simulink model "momentTest_th"  (R2018b)
settings: Solver=ode3  StartTime=0.0  StopTime=sim_time  FixedStep=.001  RelTol=1e-3
values from neighbouring files (symbols this model uses):
  accMag = tetherTen/mass    (= 25.8815917179)    [momentTest_ts.m]
  initPos = [path_init(1);path_init(2);path_init(3);]    [momentTest_ts.m]
  initVelTan = velMag*[cosd(initVelAng);sind(initVelAng);0]    [momentTest_ts.m]
  MOI_X = 1e5    (= 100000)    [momentTest_ts.m]
libraries: schmehlTangentRotation_ul x1, vectorNormalizer_ul x1, pathFollowingController_cl x1
settings Model: Creator=jldanie5  LastModifiedBy=jldanie5
settings DebuggingCC: BusObjectLabelMismatch=none  UnderSpecifiedDimensionMsg=warning

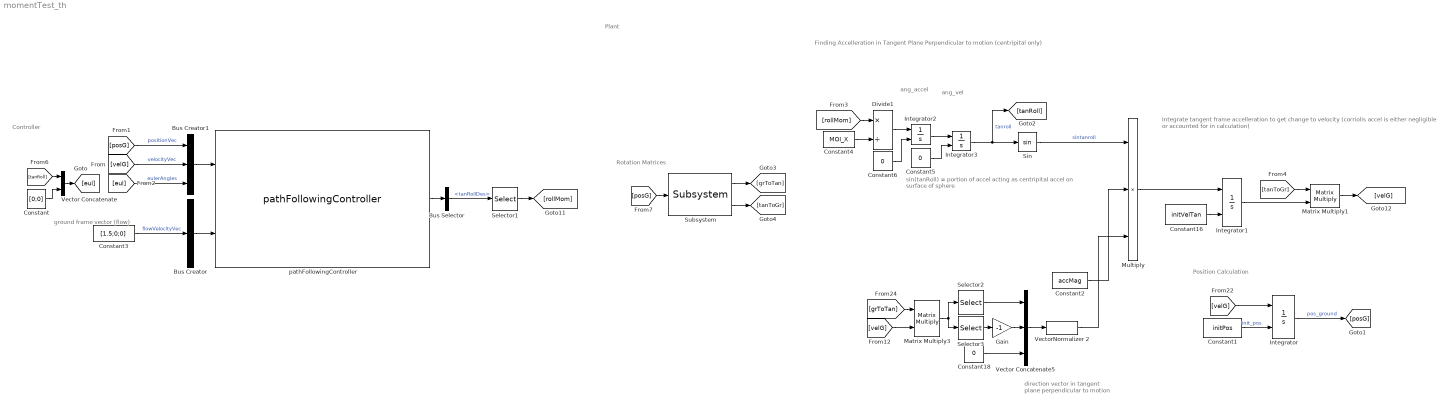
== system momentTest_th ==
  note: ground frame
      | vector (flow)
  note: Rotation Matrices
  note: Controller
  note: Integrate tangent frame accelleration to get change to
      | velocity (corriolis accel is either negligible or accounted for
      | in calculation)
  note: Finding Accelleration in Tangent Plane Perpendicular to motion (centripital only)
  note: ang_vel
  note: ang_accel
  note: sin(tanRoll) = portion of accel acting as centripital accel
      | on surface of sphere
  note: direction vector in tangent
      | plane perpendicular to motion
  note: Position Calculation
  note: Plant
  Bus Creator : BusCreator  Inputs=1  OutDataTypeStr=Bus: envBus
      settings: InheritFromInputs=off
  Bus Creator1 : BusCreator  Inputs=3  OutDataTypeStr=Bus: plantBus
  Bus Selector : BusSelector  OutputSignals=tanRollDes
  Constant : Constant  Value=[0;0]  VectorParams1D=off
  Constant1 : Constant  Value=initPos
  Constant16 : Constant  Value=initVelTan
  Constant18 : Constant  Value=0
  Constant2 : Constant  Value=accMag
  Constant3 : Constant  Value=[1.5;0;0]
  Constant4 : Constant  Value=MOI_X
  Constant5 : Constant  Value=0
  Constant6 : Constant  Value=0
  Divide1 : Product  Inputs=*/
  Gain : Gain  Gain=-1
  Integrator{,1..3} (4 alike) : Integrator  InitialConditionSource=external
  Matrix Multiply1 : Product  Multiplication=Matrix(*)
  Matrix Multiply3 : Product  Multiplication=Matrix(*)
  Multiply : Product  Inputs=3
  Selector1 : Selector  InputPortWidth=3  IndexOptions=Index vector (dialog)  Indices=1  OutputSizes=1
  Selector2 : Selector  InputPortWidth=3  IndexOptions=Index vector (dialog)  Indices=2  OutputSizes=1
  Selector3 : Selector  InputPortWidth=3  IndexOptions=Index vector (dialog)  Indices=1  OutputSizes=1
  Sin : Trigonometry
  Subsystem : schmehlTangentRotation_ul/Subsystem  SystemSampleTime=-1
  Vector Concatenate : Concatenate
  Vector Concatenate5 : Concatenate  NumInputs=3
  VectorNormalizer 2 : vectorNormalizer_ul/VectorNormalizer   SystemSampleTime=-1
  pathFollowingController : pathFollowingController_cl/pathFollowingController  initPosForInitSStar=initPos  searchSizeMask=pi/4  curveLatMask=latCurve  aMask=aBooth  bMask=bBooth  perpErrorValMask=3*pi/180  controlSigMaxMask=controlSigMax  maxBankMask=maxBank  controlAlMatMask=controlAlMat  kpVelAngMask=kpVelAng  kdVelAngMask=kdVelAng  tauVelAngMask=tauVelAng  kpLMask=kpRollMom  kdLMask=kdRollMom  tauLMask=tauRollMom
  wires:
  Constant1/1 -> Integrator/2  "init_pos"
  Integrator/1 -> [posG]  "pos_ground"
  [posG] -> Bus Creator1/1  "positionVec"
  [velG] -> Bus Creator1/2  "velocityVec"
  [eul] -> Bus Creator1/3  "eulerAngles"
  Bus Creator1/1 -> pathFollowingController/1
  [posG] -> Subsystem/1
  Subsystem/1 -> [grToTan]
  Subsystem/2 -> [tanToGr]
  [velG] -> Integrator/1
  [velG] -> Matrix Multiply3/2
  [grToTan] -> Matrix Multiply3/1
  Matrix Multiply3/1 -> Selector3/1, Selector2/1
  Selector2/1 -> Vector Concatenate5/1
  Constant16/1 -> Integrator1/2
  Constant18/1 -> Vector Concatenate5/3
  Multiply/1 -> Integrator1/1
  Selector3/1 -> Gain/1
  Gain/1 -> Vector Concatenate5/2
  Integrator3/1 -> Sin/1, [tanRoll]  "tanroll"
  VectorNormalizer 2/1 -> Multiply/3
  Vector Concatenate5/1 -> VectorNormalizer 2/1
  Constant2/1 -> Multiply/2
  Integrator2/1 -> Integrator3/1
  [rollMom] -> Divide1/1
  Divide1/1 -> Integrator2/1
  Constant4/1 -> Divide1/2
  Constant5/1 -> Integrator3/2
  Constant6/1 -> Integrator2/2
  Sin/1 -> Multiply/1  "sintanroll"
  Matrix Multiply1/1 -> [velG]
  [tanToGr] -> Matrix Multiply1/1
  Integrator1/1 -> Matrix Multiply1/2
  pathFollowingController/1 -> Bus Selector/1
  Bus Selector/1 -> Selector1/1  "<tanRollDes>"
  Selector1/1 -> [rollMom]
  Bus Creator/1 -> pathFollowingController/2
  Constant3/1 -> Bus Creator/1  "flowVelocityVec"
  [tanRoll] -> Vector Concatenate/1
  Constant/1 -> Vector Concatenate/2
  Vector Concatenate/1 -> [eul]
